simulink model "statecontrol1"  (R2022b)
settings: Solver=VariableStepAuto  StartTime=0.0  StopTime=5  RelTol=1e-3
model workspace (MAT data in the model file):
  CC = [-1 -1]
values from neighbouring files (symbols this model uses):
  A = [-5 2 3 0 0 0 ... (first row only)    [retest004.m]    (also in retest007.m = [0	1	0	0)
  Bru = eye(6)    [retest004.m]    (also in retest007.m = [1.30358515621439e-08	1.30358515745248e-08)
  C = [1,0,0,0,0,0]    [retest004.m]    (also in retest007.m = [16.0376601050147	0.425434196872911	-35.4185444812321	-0.584)
  U0 = wa_0    [retest004.m]    (also in retest007.m)
undefined symbols (not defined in the file or in its folder): sigbuilder_block
libraries: simulink x1
settings Model: Creator=Administrator  LastModifiedBy=NINGMEI

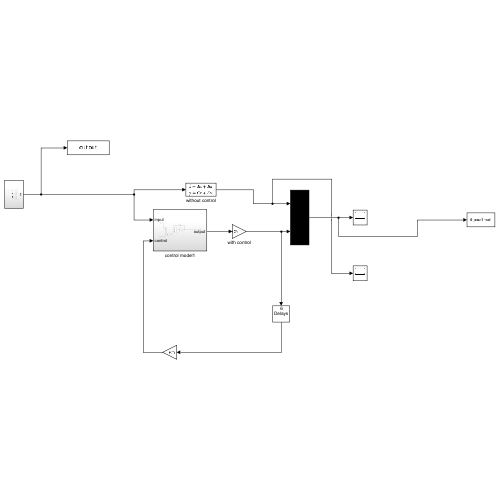
[thumbnail: Simulink's stored preview of the top-level diagram]
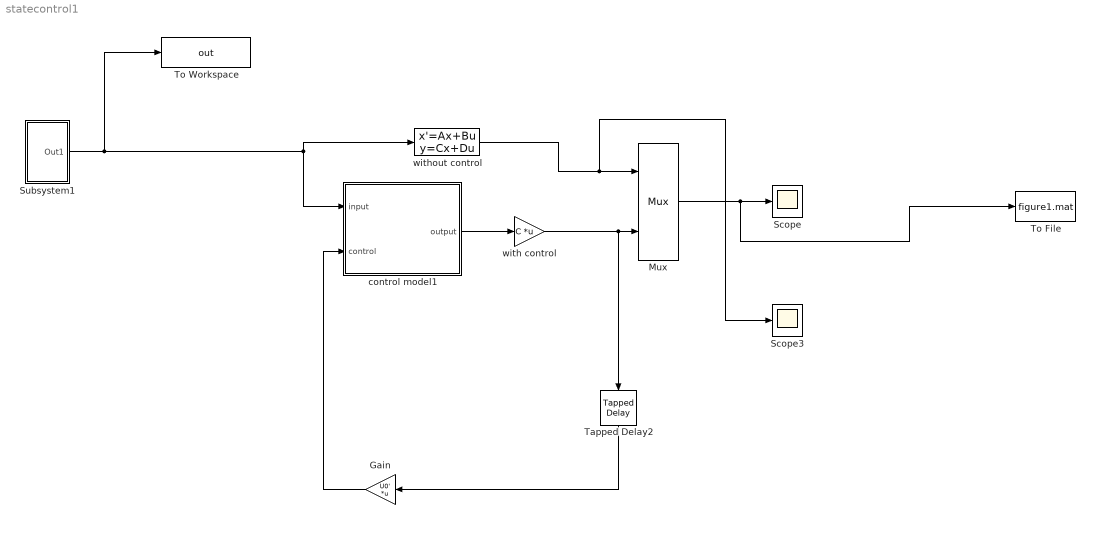
== system statecontrol1 ==
  Gain : Gain  Gain=U0'  Multiplication=Matrix(K*u)
  Mux : Mux  Inputs=2
  Scope : Scope
  Scope3 : Scope
  Subsystem1 : Subsystem
  Tapped Delay2 : simulink/Discrete/Tapped Delay  vinit=0.0  samptime=0.00025  NumDelays=6  DelayOrder=Oldest  includeCurrent=off
  To File : ToFile  Filename=figure1.mat  SaveFormat=Timeseries
  To Workspace : ToWorkspace  VariableName=out  SaveFormat=Timeseries  SampleTime=-1
  control model1 : Subsystem
  with control : Gain  Gain=C  Multiplication=Matrix(K*u)
  without control : StateSpace  A=A  B=Bru  C=C  D=zeros(1,6)  InitialCondition=0
  wires:
  without control/1 -> Scope3/1, Mux/1
  Gain/1 -> control model1/2(control)
  Mux/1 -> To File/1, Scope/1
  control model1/1(output) -> with control/1
  with control/1 -> Mux/2, Tapped Delay2/1
  Tapped Delay2/1 -> Gain/1
  Subsystem1/1(Out1) -> To Workspace/1, without control/1, control model1/1(input)

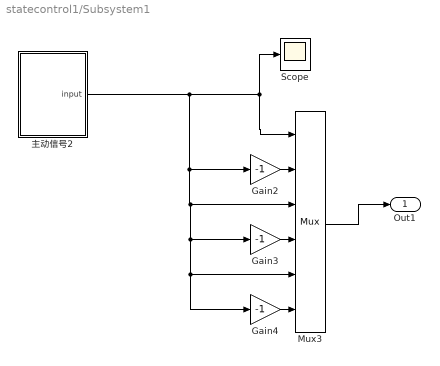
== system statecontrol1/Subsystem1 ==
  Gain2 : Gain  Gain=-1
  Gain3 : Gain  Gain=-1
  Gain4 : Gain  Gain=-1
  Mux3 : Mux  Inputs=6
  Scope : Scope
  主动信号2 : Subsystem
  Out1 : Outport
  wires:
  Mux3/1 -> Out1/1
  Gain2/1 -> Mux3/2
  Gain3/1 -> Mux3/4
  Gain4/1 -> Mux3/6
  主动信号2/1(input) -> Gain4/1, Mux3/5, Gain3/1, Mux3/3, Gain2/1, Mux3/1, Scope/1

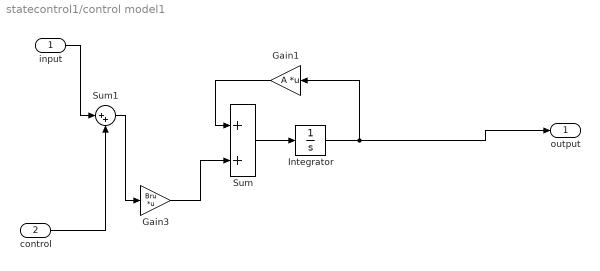
== system statecontrol1/control model1 ==
  input : Inport
  control : Inport  Port=2
  Gain1 : Gain  Gain=A  Multiplication=Matrix(K*u)
  Gain3 : Gain  Gain=Bru  Multiplication=Matrix(K*u)
  Integrator : Integrator
  Sum : Sum  Inputs=|++
  Sum1 : Sum  Inputs=|++
  output : Outport
  wires:
  Gain1/1 -> Sum/1
  Sum/1 -> Integrator/1
  Gain3/1 -> Sum/2
  Integrator/1 -> output/1, Gain1/1
  input/1 -> Sum1/1
  control/1 -> Sum1/2
  Sum1/1 -> Gain3/1

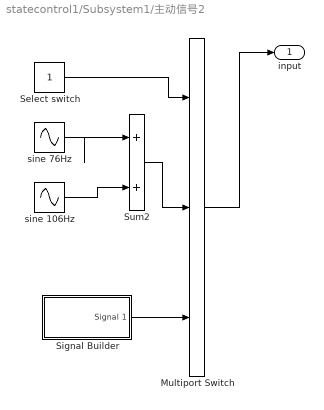
== system statecontrol1/Subsystem1/主动信号2 ==
  Multiport Switch : MultiPortSwitch  Inputs=2  SaturateOnIntegerOverflow=off  InputSameDT=off
  Select switch : Constant
  Signal Builder : Subsystem  Tag=STV Subsys  LoadFcn=sigbuilder_block('load');  StartFcn=sigbuilder_block('start');  StopFcn=sigbuilder_block('stop');  ClipboardFcn=sigbuilder_block('clipboard');  mask(Sigbuilder block){tuvar=[0:10]}
      mask help: Simulink:masks:SigbuilderBlock_MD
      mask init:
      | if ~strcmp(get_param(bdroot(gcbh),'SimulationStatus'),'stopped') tuvar = sigbuilder_block('maskInit'); end
      settings: CopyFcn=sigbuilder_block('copy');  DeleteFcn=sigbuilder_block('delete');  ModelCloseFcn=sigbuilder_block('modelClose');  PreSaveFcn=sigbuilder_block('preSave');  PauseFcn=sigbuilder_block('pause');  ContinueFcn=sigbuilder_block('continue');  NameChangeFcn=sigbuilder_block('namechange');  OpenFcn=sigbuilder_block('open',[230.897 85.6552 549.931 396.621 ]);  CloseFcn=sigbuilder_block('close');
      mask Display: plot(0, 0, 100, 100,[2, 2, 32, 32, 2], [68, 8, 8, 68, 68],[32, 2], [38, 38], [32, 19, 2],[53, 60, 44], [32, 17, 17, 2],[16, 16, 31, 31]);txt = getActiveGroup(gcbh);text(2, 100, txt,'verticalAlignment', 'top');
  Sum2 : Sum  Inputs=|++
  sine 106Hz : Sin  Amplitude=5  Frequency=2*pi*1.06  SampleTime=0
  sine 76Hz : Sin  Amplitude=5  Frequency=2*pi*0.76  SampleTime=0
  input : Outport
  wires:
  Select switch/1 -> Multiport Switch/1
  sine 76Hz/1 -> Sum2/1
  Multiport Switch/1 -> input/1
  Signal Builder/1(Signal 1) -> Multiport Switch/3
  sine 106Hz/1 -> Sum2/2
  Sum2/1 -> Multiport Switch/2

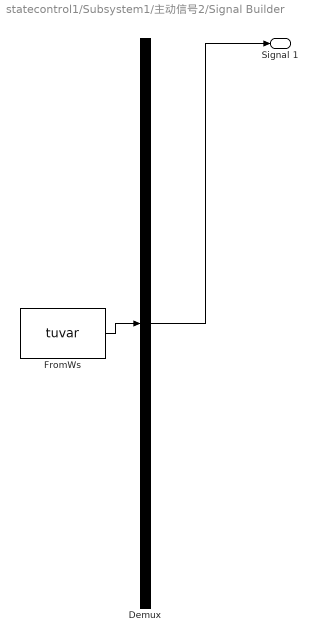
== system statecontrol1/Subsystem1/主动信号2/Signal Builder ==
  Demux : Demux  Tag=STV Demux  Outputs=1
      settings: DisplayOption=none
  FromWs : FromWorkspace  Tag=STV FromWs  VariableName=tuvar
      SigBuilderData=|
      | common.afterFinalStr = 'Extrapolate'
      | common.sampleTime = 0
      | dataSet.timeRange = [0 10]
      | dataSet.name = 'Group 1'
      | sbobj.Groups.Name = 'Group 1'
      | sbobj.Groups.Signals.Name = 'Signal 1'
      | sbobj.Groups.Signals.XData = [0 0.1 0.1 0.1001 0.1001 10]
      | sbobj.Groups.Signals.YData = [0 0 1 1 0 0]
  Signal 1 : Outport  Tag=STV Outport
  wires:
  Demux/1 -> Signal 1/1
  FromWs/1 -> Demux/1
